simulink model "reaction_wheels_nonlinear_v03"  (R2015b)
settings: Solver=VariableStepAuto  StartTime=0.0  StopTime=stop_time  RelTol=1e-6
values from neighbouring files (symbols this model uses):
  B_quaternion = [zeros(4,3);diag([1/I_x 1/I_y 1/I_z])]    [main_reaction_wheels_detumbling.m]    (also in main_reaction_wheels_nonlinear_v03.m)
  I_x = 1    [main_linear_spacecraft_euler.m]    (also in main_reaction_nonlinear_v02.m; main_reaction_wheels_detumbling.m; main_reaction_wheels_nonlinear_v01.m; main_reaction_wheels_nonlinear_v03.m)
  I_y = 0.5    [main_linear_spacecraft_euler.m]    (also in main_reaction_nonlinear_v02.m; main_reaction_wheels_detumbling.m; main_reaction_wheels_nonlinear_v01.m; main_reaction_wheels_nonlinear_v03.m)
  I_z = 0.7    [main_linear_spacecraft_euler.m]    (also in main_reaction_nonlinear_v02.m; main_reaction_wheels_detumbling.m; main_reaction_wheels_nonlinear_v01.m; main_reaction_wheels_nonlinear_v03.m)
  k_d = 4    [main_pd_control.m]    (also in main_reaction_nonlinear_v02.m = 2*zeta_0*omega_n_0*I_max; main_reaction_wheels_nonlinear_v03.m = 2*zeta_0*omega_n_0*I_max)
  k_p = 9    [main_pd_control.m]    (also in main_reaction_nonlinear_v02.m = 2*omega_n_0^2*I_max; main_reaction_wheels_nonlinear_v03.m = 2*omega_n_0^2*I_max)
  x_0 = [phi_0 ... (first row only)    [main_linear_spacecraft_euler.m]    (also in main_reaction_wheels_detumbling.m = [epsilon_0; main_reaction_wheels_nonlinear_v03.m = [epsilon_0)
settings Model: Creator=Krunal's PC  LastModifiedBy=Krunal's PC

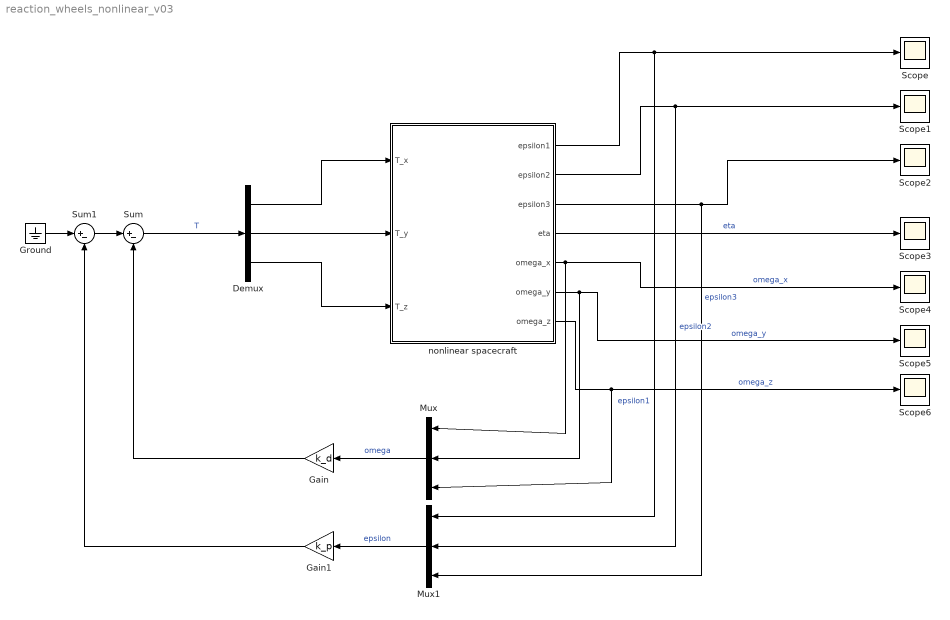
== system reaction_wheels_nonlinear_v03 ==
  Demux : Demux  Outputs=3
  Gain : Gain  Gain=k_d
  Gain1 : Gain  Gain=k_p
  Ground : Ground
  Mux : Mux  Inputs=3
  Mux1 : Mux  Inputs=3
  Scope{,1..6} (7 alike) : Scope
  Sum : Sum  Inputs=|+-
  Sum1 : Sum  Inputs=|+-
  nonlinear spacecraft : Subsystem
  wires:
  nonlinear spacecraft/1(epsilon1) -> Mux1/1, Scope/1  "epsilon1"
  nonlinear spacecraft/2(epsilon2) -> Mux1/2, Scope1/1  "epsilon2"
  nonlinear spacecraft/3(epsilon3) -> Mux1/3, Scope2/1  "epsilon3"
  nonlinear spacecraft/4(eta) -> Scope3/1  "eta"
  nonlinear spacecraft/5(omega_x) -> Scope4/1, Mux/1  "omega_x"
  nonlinear spacecraft/6(omega_y) -> Mux/2, Scope5/1  "omega_y"
  nonlinear spacecraft/7(omega_z) -> Mux/3, Scope6/1  "omega_z"
  Mux/1 -> Gain/1  "omega"
  Mux1/1 -> Gain1/1  "epsilon"
  Demux/2 -> nonlinear spacecraft/2(T_y)
  Demux/1 -> nonlinear spacecraft/1(T_x)
  Demux/3 -> nonlinear spacecraft/3(T_z)
  Gain/1 -> Sum/2
  Sum/1 -> Demux/1  "T"
  Sum1/1 -> Sum/1
  Gain1/1 -> Sum1/2
  Ground/1 -> Sum1/1

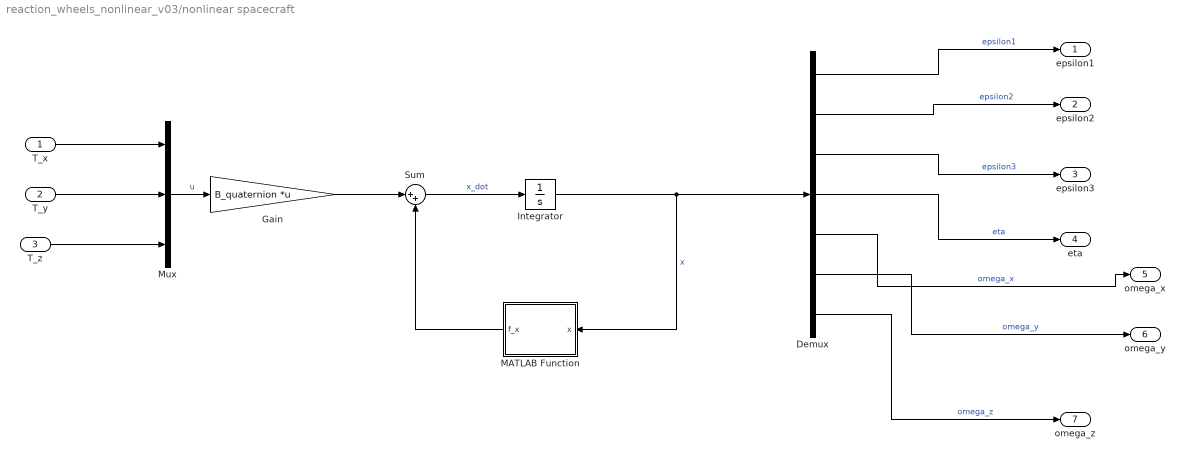
== system reaction_wheels_nonlinear_v03/nonlinear spacecraft ==
  T_x : Inport
  T_y : Inport  Port=2
  T_z : Inport  Port=3
  Demux : Demux  Outputs=7
  Gain : Gain  Gain=B_quaternion  Multiplication=Matrix(K*u)
  Integrator : Integrator  InitialCondition=x_0
  MATLAB Function : MATLAB Function  TreatAsAtomicUnit=on
  Mux : Mux  Inputs=3
  Sum : Sum  Inputs=|++
  epsilon1 : Outport
  epsilon2 : Outport  Port=2
  epsilon3 : Outport  Port=3
  eta : Outport  Port=4
  omega_x : Outport  Port=5
  omega_y : Outport  Port=6
  omega_z : Outport  Port=7
  wires:
  T_z/1 -> Mux/3
  Integrator/1 -> MATLAB Function/1(x), Demux/1  "x"
  T_y/1 -> Mux/2
  T_x/1 -> Mux/1
  Mux/1 -> Gain/1  "u"
  Gain/1 -> Sum/1
  Sum/1 -> Integrator/1  "x_dot"
  MATLAB Function/1(f_x) -> Sum/2
  Demux/1 -> epsilon1/1  "epsilon1"
  Demux/2 -> epsilon2/1  "epsilon2"
  Demux/3 -> epsilon3/1  "epsilon3"
  Demux/4 -> eta/1  "eta"
  Demux/5 -> omega_x/1  "omega_x"
  Demux/6 -> omega_y/1  "omega_y"
  Demux/7 -> omega_z/1  "omega_z"

== matlab function reaction_wheels_nonlinear_v03/nonlinear spacecraft/MATLAB Function ==
  data: x input; f_x output; I_x parameter; I_y parameter; I_z parameter
function f_x = fcn(x,I_x,I_y,I_z)
epsilon=zeros(3,1);

epsilon(1,1)=x(1);
epsilon(2,1)=x(2);
epsilon(3,1)=x(3);
eta=x(4);
omega_x=x(5);
omega_y=x(6);
omega_z=x(7);
omega=[omega_x;omega_y;omega_z];
epsilon_cross=[0 -epsilon(3,1) epsilon(2,1);
               epsilon(3,1) 0 -epsilon(1,1);
               -epsilon(2,1) epsilon(1,1) 0];
           
epsilon_dot=1/2*(eta*eye(3)+epsilon_cross)*omega;           
eta_dot= -1/2*epsilon'*omega;
f_x=zeros(7,1);

f_x(1,1)= epsilon_dot(1,1);
f_x(2,1)= epsilon_dot(2,1);
f_x(3,1)= epsilon_dot(3,1);
f_x(4,1)=eta_dot
f_x(5,1)=(I_y-I_z)/I_x*(omega_y*omega_z);
f_x(6,1)=(I_z-I_x)/I_y*(omega_x*omega_z);
f_x(7,1)=(I_x-I_y)/I_z*(omega_x*omega_y);
